simulink model "Machine"  (R2025a)
settings: Solver=VariableStepAuto  StartTime=0.0  StopTime=10  RelTol=1e-3
settings Model: Creator=cruisemac  LastModifiedBy=cruisemac

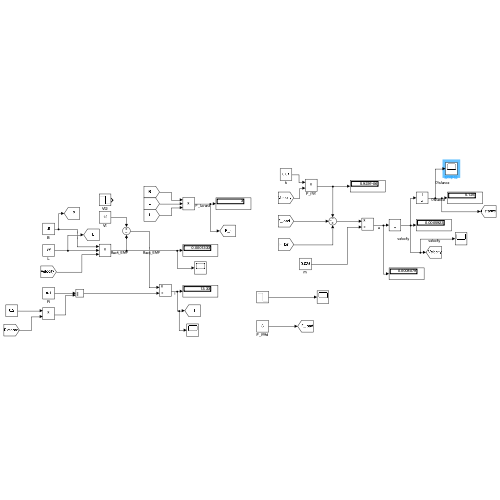
[thumbnail: Simulink's stored preview of the top-level diagram]
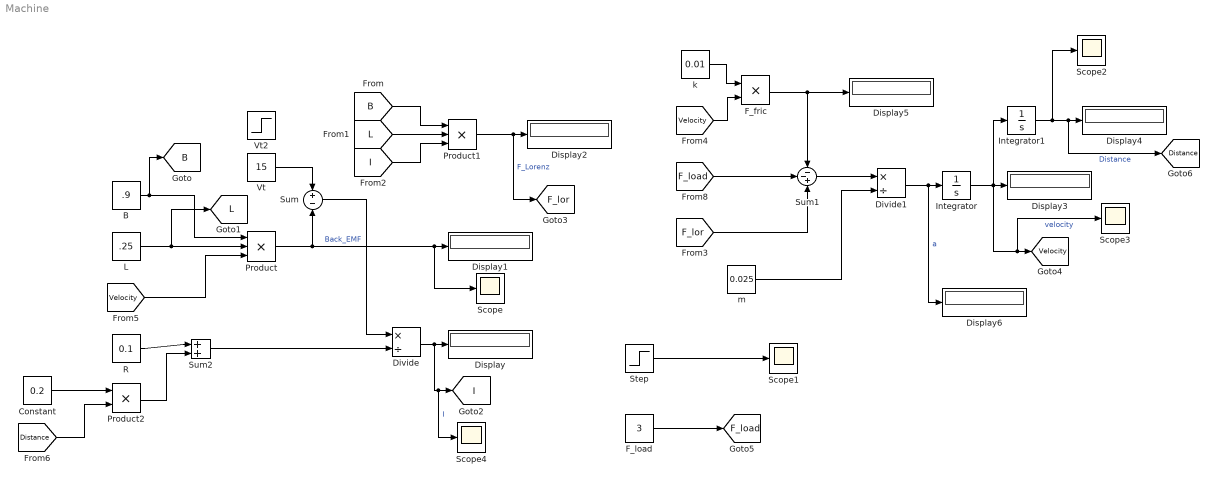
== system Machine ==
  B : Constant  Value=.9
  Constant : Constant  Value=0.2
  Display{,1..6} (7 alike) : Display
  Divide : Product  Inputs=*/
  Divide1 : Product  Inputs=*/
  F_fric : Product
  F_load : Constant  Value=3
  Integrator : Integrator
  Integrator1 : Integrator
  L : Constant  Value=.25
  Product : Product  Inputs=3
  Product1 : Product  Inputs=3
  Product2 : Product
  R : Constant  Value=0.1
  Scope{,1..4} (5 alike) : Scope
      Scope settings: ActiveDisplayYMinimum=-4.3904835887443259  ActiveDisplayYMaximum=7.8714409572303357
      Scope1 settings: ActiveDisplayYMinimum=-1  ActiveDisplayYMaximum=1
      Scope2 settings: ActiveDisplayYMinimum=-1.2959539919313374  ActiveDisplayYMaximum=11.663585927382039  DataLoggingVariableName=ScopeData2
      Scope3 settings: ActiveDisplayYMinimum=-19.513260394419227  ActiveDisplayYMaximum=34.984182032134825  DataLoggingVariableName=ScopeData3
      Scope4 settings: ActiveDisplayYMinimum=-11.670623666806463  ActiveDisplayYMaximum=167.96340262964517  DataLoggingVariableName=ScopeData4
  Step : Step  Before=3  After=-5  SampleTime=0
  Sum : Sum  Inputs=+-
  Sum1 : Sum  Inputs=--+
  Sum2 : Sum  Inputs=|++
  Vt : Constant  Value=15
  Vt2 : Step  Before=15  After=-15  SampleTime=0
  k : Constant  Value=0.01
  m : Constant  Value=0.025
  tag scope: B=global, Distance=global, F_load=global, F_lor=global, I=global, L=global, Velocity=global
  wires:
  B/1 -> [B], Product/1
  L/1 -> Product/2, [L]
  Product/1 -> Scope/1, Display1/1, Sum/2  "Back_EMF"
  Sum/1 -> Divide/1
  Divide/1 -> Scope4/1, [I], Display/1  "I"
  [B] -> Product1/1
  [L] -> Product1/2
  [I] -> Product1/3
  Product1/1 -> [F_lor], Display2/1  "F_Lorenz"
  k/1 -> F_fric/1
  [F_lor] -> Sum1/3
  [F_load] -> Sum1/2
  F_fric/1 -> Display5/1, Sum1/1
  Sum1/1 -> Divide1/1
  m/1 -> Divide1/2
  Divide1/1 -> Display6/1, Integrator/1  "a"
  Integrator/1 -> Integrator1/1, Scope3/1, [Velocity], Display3/1  "velocity"
  [Velocity] -> F_fric/2
  [Velocity] -> Product/3
  Integrator1/1 -> Scope2/1, [Distance], Display4/1  "Distance"
  Step/1 -> Scope1/1
  F_load/1 -> [F_load]
  [Distance] -> Product2/2
  Constant/1 -> Product2/1
  R/1 -> Sum2/1
  Product2/1 -> Sum2/2
  Sum2/1 -> Divide/2
  Vt/1 -> Sum/1
